simulink model "FOC_FZ"  (R2023b)
settings: Solver=FixedStepDiscrete  StartTime=0.0  StopTime=5  FixedStep=0.000001  RelTol=1e-3
libraries: simulink x2, spsDCVoltageSourceLib x1, spsPermanentMagnetSynchronousMachineLib x1, spsTwoLevelConverterLib x1, sps_lib x1
settings Model: Creator=LQY  LastModifiedBy=LQY

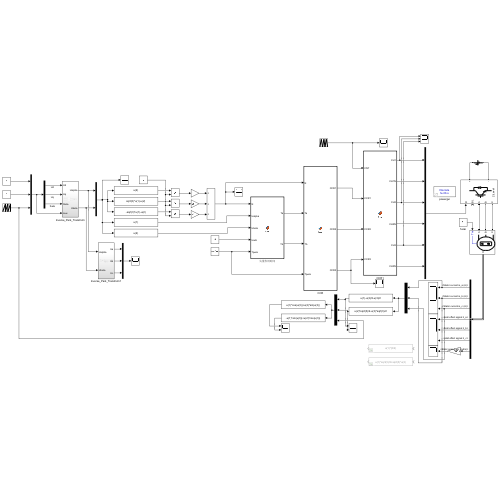
[thumbnail: Simulink's stored preview of the top-level diagram]
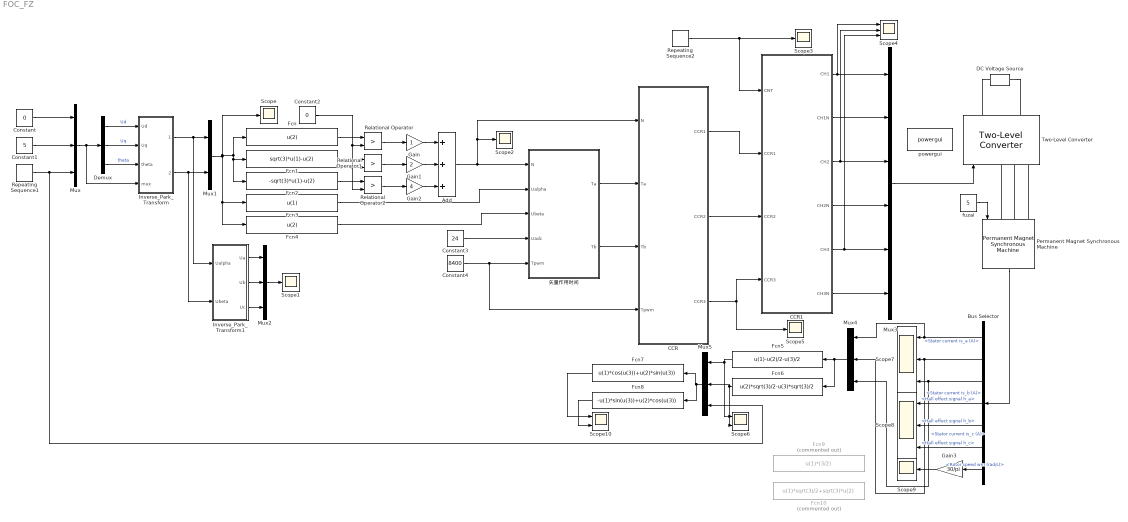
== system FOC_FZ ==
  Add : Sum  Inputs=+++
  Bus Selector : BusSelector  OutputSignals=Stator current is_a (A),Stator current is_b (A),Stator current is_c (A),Hall effect signal h_a,Hall effect signal h_b,Hall effect signal h_c,Rotor speed wm (rad/s)
  CCR : MATLAB Function  TreatAsAtomicUnit=on
  CCR1 : MATLAB Function  TreatAsAtomicUnit=on
  Constant : Constant  Value=0
  Constant1 : Constant  Value=5
  Constant2 : Constant  Value=0
  Constant3 : Constant  Value=24
  Constant4 : Constant  Value=8400
  DC Voltage Source : spsDCVoltageSourceLib/DC Voltage Source  Amplitude=24  Measurements=None
  Demux : Demux  Outputs=3
  Fcn : Fcn  Expr=u(2)
  Fcn1 : Fcn  Expr=sqrt(3)*u(1)-u(2)
  Fcn10 : Fcn  Commented=on  Expr=u(1)*sqrt(3)/2+sqrt(3)*u(2)
  Fcn2 : Fcn  Expr=-sqrt(3)*u(1)-u(2)
  Fcn3 : Fcn  Expr=u(1)
  Fcn4 : Fcn  Expr=u(2)
  Fcn5 : Fcn  Expr=u(1)-u(2)/2-u(3)/2
  Fcn6 : Fcn  Expr=u(2)*sqrt(3)/2-u(3)*sqrt(3)/2
  Fcn7 : Fcn  Expr=u(1)*cos(u(3))+u(2)*sin(u(3))
  Fcn8 : Fcn  Expr=-u(1)*sin(u(3))+u(2)*cos(u(3))
  Fcn9 : Fcn  Commented=on  Expr=u(1)*(3/2)
  Gain : Gain
  Gain1 : Gain  Gain=2
  Gain2 : Gain  Gain=4
  Gain3 : Gain  Gain=30/pi
  Inverse_Park_Transform : Subsystem
  Inverse_Park_Transform1 : Subsystem
  Mux{,2,4..5} (4 alike) : Mux  Inputs=3
  Mux1 : Mux  Inputs=2
  Mux3 : Mux  Inputs=6
  Permanent Magnet Synchronous Machine : spsPermanentMagnetSynchronousMachineLib/Permanent Magnet Synchronous Machine  NbPhases=3  FluxDistribution=Sinusoidal  RotorType=Round  MechanicalLoad=Torque Tm  PresetModel=No  ShowDetailedParameters=on  MeasurementBus=off  Resistance=0.0485  Inductance=8.5e-3  dqInductances=[8.5e-3,8.5e-3]  La=0.000395  MachineConstant=Flux linkage established by magnets (V.s)  Flux=0.1194  VoltageCst=43.3135  TorqueCst=0.3582  Flat=120  Mechanical=[0.0027 0.0004924 2 0]  PolePairs=4  InitialConditions=[0,0, 0,0]  InitialConditions5ph=[0 0 0 0 0 0]  RefAngle=Aligned with phase A axis (original Park)  IterativeDiscreteModel=Trapezoidal non iterative  TsBlock=-1  TsPowergui=0
  Relational Operator : RelationalOperator  Operator=>  OutDataTypeStr=boolean  RndMeth=Simplest  InputSameDT=off
  Relational Operator1 : RelationalOperator  Operator=>  OutDataTypeStr=boolean  RndMeth=Simplest  InputSameDT=off
  Relational Operator2 : RelationalOperator  Operator=>  OutDataTypeStr=boolean  RndMeth=Simplest  InputSameDT=off
  Repeating Sequence1 : simulink/Sources/Repeating Sequence  rep_seq_t=[0 0.5]  rep_seq_y=[0 2*pi]
  Repeating Sequence2 : simulink/Sources/Repeating Sequence  rep_seq_t=[0 0.00005 0.0001]  rep_seq_y=[0 4200 0]
  Scope{,1..3,5,9} (6 alike) : Scope
  Scope10 : Scope  NumInputPorts=2
  Scope4 : Scope  NumInputPorts=3
  Scope6 : Scope  NumInputPorts=2
  Scope7 : Scope  NumInputPorts=3
  Scope8 : Scope  NumInputPorts=3
  Two-Level Converter : spsTwoLevelConverterLib/Two-Level Converter  ModelType=Switching devices  Ron=1e-3  Rs=1e6  Cs=inf  Vforward=[0,0]  Ron_Diode=1e-3  Rs_Diode=1e6  Cs_Diode=inf  Vf_Diode=1e-3  Rs_CurrentSource=inf  Ron_ACsource=1e-3
      settings: LibrarySourceBlock=sps_lib/Power Electronics/Two-Level Converter
  fuzai : Constant  Value=5
  powergui : sps_lib/powergui  Priority=1  SimulationMode=Discrete  SampleTime=0.000001  frequency=60  Iterations=50  frequencyindice=0  Pbase=100e6  ErrMax=1e-4  UnitsV=kV  UnitsW=MW  buscounter=0  FunctionMessages=off  echomessages=off  EnableUseOfTLC=off  CurrentSourceSwitches=off  DisableSnubberDevices=off  DisableRonSwitches=off  DisableVfSwitches=off  DisplayEquations=off  AutomaticDiscreteSolvers=off  SolverType=Tustin/Backward Euler (TBE)  Interpol=off  ExternalGateDelay=off  methode=off  Ts=100  x0status=blocks  SPID=on  SwTol=0  HookPort=off  NonlinearTolerance=1e-4  nMaxIteration=100  ContinueOnMaxIteration=off  RestoreLinks=warning  ResistiveCurrentMeasurement=off  Frange=[0:2:500]  Ylog=off  Xlog=on  ShowGrid=off  save=off  variable=ZData  structure=0  ZoomFFT=off  StartTime=0.0  cycles=1  DisplayStyle=1  fundamental=60  FreqAxis=off  MaxFrequency=1000  frequencyindicesteady=1  RmsSteady=1  display=off
  矢量作用时间 : MATLAB Function  TreatAsAtomicUnit=on
  wires:
  Constant/1 -> Mux/1
  Constant1/1 -> Mux/2
  Repeating Sequence1/1 -> Mux5/3, Mux/3
  Mux/1 -> Inverse_Park_Transform/4(mux), Demux/1
  Mux1/1 -> Fcn2/1, Fcn1/1, Fcn/1, Scope/1, Fcn4/1, Fcn3/1
  Demux/1 -> Inverse_Park_Transform/1(Ud)  "Ud"
  Demux/2 -> Inverse_Park_Transform/2(Uq)  "Uq"
  Demux/3 -> Inverse_Park_Transform/3(theta)  "theta"
  Inverse_Park_Transform/1(Ualpha) -> Inverse_Park_Transform1/1(Ualpha), Mux1/1
  Inverse_Park_Transform/2(Ubeta) -> Mux1/2, Inverse_Park_Transform1/2(Ubeta)
  Inverse_Park_Transform1/2(Ub) -> Mux2/2
  Inverse_Park_Transform1/1(Ua) -> Mux2/1
  Inverse_Park_Transform1/3(Uc) -> Mux2/3
  Mux2/1 -> Scope1/1
  Fcn/1 -> Relational Operator/1
  Constant2/1 -> Relational Operator/2, Relational Operator1/2, Relational Operator2/2
  Fcn1/1 -> Relational Operator1/1
  Fcn2/1 -> Relational Operator2/1
  Relational Operator/1 -> Gain/1
  Relational Operator1/1 -> Gain1/1
  Relational Operator2/1 -> Gain2/1
  Gain/1 -> Add/1
  Gain1/1 -> Add/2
  Gain2/1 -> Add/3
  Add/1 -> 矢量作用时间/1(N), CCR/1(N), Scope2/1
  Fcn3/1 -> 矢量作用时间/2(Ualpha)
  Fcn4/1 -> 矢量作用时间/3(Ubeta)
  Constant3/1 -> 矢量作用时间/4(Uadc)
  Constant4/1 -> CCR/4(Tpwm), 矢量作用时间/5(Tpwm)
  矢量作用时间/1(Ta) -> CCR/2(Ta)
  矢量作用时间/2(Tb) -> CCR/3(Tb)
  Repeating Sequence2/1 -> CCR1/1(CNT), Scope3/1
  CCR/1(CCR1) -> CCR1/2(CCR1)
  CCR/2(CCR2) -> CCR1/3(CCR2)
  CCR/3(CCR3) -> Scope5/1, CCR1/4(CCR3)
  CCR1/6(CH3N) -> Mux3/6
  CCR1/5(CH3) -> Scope4/3, Mux3/5
  CCR1/4(CH2N) -> Mux3/4
  CCR1/3(CH2) -> Scope4/2, Mux3/3
  CCR1/2(CH1N) -> Mux3/2
  CCR1/1(CH1) -> Scope4/1, Mux3/1
  Mux3/1 -> Two-Level Converter/1
  fuzai/1 -> Permanent Magnet Synchronous Machine/1
  Permanent Magnet Synchronous Machine/1 -> Bus Selector/1
  Bus Selector/1 -> Mux4/1, Scope7/1  "<Stator current is_a (A)>"
  Bus Selector/2 -> Mux4/2, Scope7/2  "<Stator current is_b (A)>"
  Bus Selector/3 -> Mux4/3, Scope7/3  "<Stator current is_c (A)>"
  Bus Selector/4 -> Scope8/1  "<Hall effect signal h_a>"
  Bus Selector/5 -> Scope8/2  "<Hall effect signal h_b>"
  Bus Selector/6 -> Scope8/3  "<Hall effect signal h_c>"
  Bus Selector/7 -> Gain3/1  "<Rotor speed wm (rad/s)>"
  Gain3/1 -> Scope9/1
  Mux4/1 -> Fcn6/1, Fcn5/1
  Fcn5/1 -> Scope6/1, Mux5/1
  Fcn6/1 -> Scope6/2, Mux5/2
  Mux5/1 -> Fcn8/1, Fcn7/1
  Fcn7/1 -> Scope10/1
  Fcn8/1 -> Scope10/2
  connections:
  DC Voltage Source/RConn1 -- Two-Level Converter/RConn1
  DC Voltage Source/LConn1 -- Two-Level Converter/RConn2
  Permanent Magnet Synchronous Machine/LConn1 -- Two-Level Converter/LConn1
  Permanent Magnet Synchronous Machine/LConn2 -- Two-Level Converter/LConn2
  Permanent Magnet Synchronous Machine/LConn3 -- Two-Level Converter/LConn3

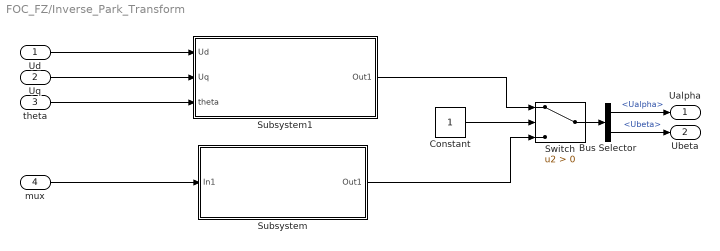
== system FOC_FZ/Inverse_Park_Transform ==
  Ud : Inport
  Uq : Inport  Port=2
  theta : Inport  Port=3
  mux : Inport  Port=4
  Bus Selector : BusSelector  OutputSignals=Ualpha,Ubeta
  Constant : Constant
  Subsystem : Subsystem
  Subsystem1 : Subsystem
  Switch : Switch  Criteria=u2 > Threshold  SaturateOnIntegerOverflow=off  InputSameDT=off
  Ualpha : Outport
  Ubeta : Outport  Port=2
  wires:
  Switch/1 -> Bus Selector/1
  Constant/1 -> Switch/2
  mux/1 -> Subsystem/1(In1)
  Subsystem/1(Out1) -> Switch/3
  Ud/1 -> Subsystem1/1(Ud)
  Uq/1 -> Subsystem1/2(Uq)
  theta/1 -> Subsystem1/3(theta)
  Subsystem1/1(Out1) -> Switch/1
  Bus Selector/2 -> Ubeta/1  "<Ubeta>"
  Bus Selector/1 -> Ualpha/1  "<Ualpha>"

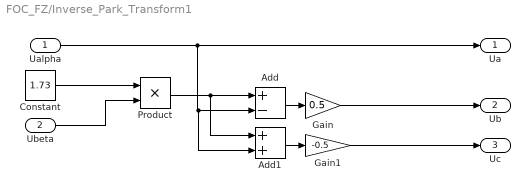
== system FOC_FZ/Inverse_Park_Transform1 ==
  Ualpha : Inport
  Ubeta : Inport  Port=2
  Add : Sum  Inputs=+-
  Add1 : Sum
  Constant : Constant  Value=1.73
  Gain : Gain  Gain=0.5
  Gain1 : Gain  Gain=-0.5
  Product : Product
  Ua : Outport
  Ub : Outport  Port=2
  Uc : Outport  Port=3
  wires:
  Ualpha/1 -> Add1/2, Add/2, Ua/1
  Constant/1 -> Product/1
  Ubeta/1 -> Product/2
  Product/1 -> Add1/1, Add/1
  Add/1 -> Gain/1
  Gain/1 -> Ub/1
  Add1/1 -> Gain1/1
  Gain1/1 -> Uc/1

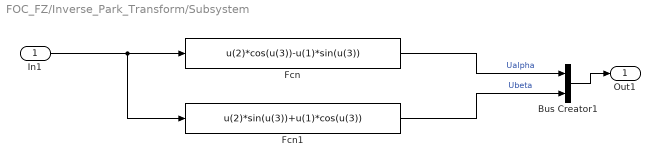
== system FOC_FZ/Inverse_Park_Transform/Subsystem ==
  In1 : Inport
  Bus Creator1 : BusCreator  Inputs=2
  Fcn : Fcn  Expr=u(2)*cos(u(3))-u(1)*sin(u(3))
  Fcn1 : Fcn  Expr=u(2)*sin(u(3))+u(1)*cos(u(3))
  Out1 : Outport
  wires:
  Fcn/1 -> Bus Creator1/1  "Ualpha"
  In1/1 -> Fcn1/1, Fcn/1
  Fcn1/1 -> Bus Creator1/2  "Ubeta"
  Bus Creator1/1 -> Out1/1

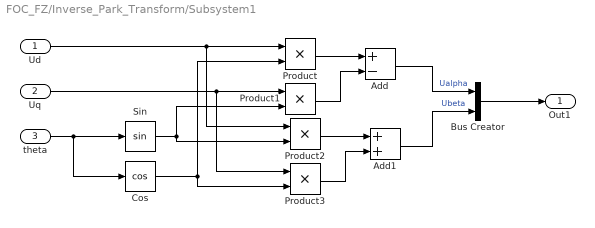
== system FOC_FZ/Inverse_Park_Transform/Subsystem1 ==
  Ud : Inport
  Uq : Inport  Port=2
  theta : Inport  Port=3
  Add : Sum  Inputs=+-
  Add1 : Sum
  Bus Creator : BusCreator  Inputs=2
  Cos : Trigonometry  Operator=cos
  Product{,1..3} (4 alike) : Product
  Sin : Trigonometry
  Out1 : Outport
  wires:
  Cos/1 -> Product3/2, Product/2
  Product3/1 -> Add1/2
  Sin/1 -> Product1/2, Product2/2
  theta/1 -> Sin/1, Cos/1
  Uq/1 -> Product3/1, Product1/1
  Ud/1 -> Product2/1, Product/1
  Product1/1 -> Add/2
  Product/1 -> Add/1
  Product2/1 -> Add1/1
  Add1/1 -> Bus Creator/2  "Ubeta"
  Add/1 -> Bus Creator/1  "Ualpha"
  Bus Creator/1 -> Out1/1

== matlab function FOC_FZ/CCR ==
  data: N input; CCR1 output; Ta input; Tb input; Tpwm input; CCR2 output; CCR3 output
function [CCR1,CCR2,CCR3] = fcn(N,Ta,Tb,Tpwm)

CCR1=double(0);
CCR2=double(0);
CCR3=double(0);

Temp=Ta+Tb;
if(Temp>Tpwm)
    Ta=Ta/Temp*Tpwm;
    Tb=Tb/Temp*Tpwm;
end

value1=(Tpwm-Ta-Tb)/4.0;
value2=value1+Ta/2.0;
value3=value2+Tb/2.0;

switch(N)
    case 3
        CCR1=value1;
        CCR2=value2;
        CCR3=value3;
    case 1
        CCR1=value2;
        CCR2=value1;
        CCR3=value3;
    case 5
        CCR1=value3;
        CCR2=value1;
        CCR3=value2;
    case 4
        CCR1=value3;
        CCR2=value2;
        CCR3=value1;
    case 6
        CCR1=value2;
        CCR2=value3;
        CCR3=value1;
    case 2
        CCR1=value1;
        CCR2=value3;
        CCR3=value2;
end

== matlab function FOC_FZ/矢量作用时间 ==
  data: N input; Ta output; Ualpha input; Ubeta input; Uadc input; Tpwm input; Tb output
function [Ta,Tb] = fcn(N,Ualpha,Ubeta,Uadc,Tpwm)

Ta=double(0);
Tb=double(0);
X=(sqrt(3)*Tpwm)/Uadc*Ubeta;            %系数1 
Y=(sqrt(3)*Tpwm)/Uadc*((sqrt(3)/2)*Ualpha-(1/2)*Ubeta);  %系数2
Z=(sqrt(3)*Tpwm)/Uadc*(-(sqrt(3)/2)*Ualpha-(1/2)*Ubeta);   %系数3
    
if(N==3)   %第一扇区
   Ta=Y;
   Tb=X;
end
if(N==1)   %第二扇区
   Ta=-Y;
   Tb=-Z;
end
if(N==5)   %第三扇区
   Ta=X;
   Tb=Z;
end
if(N==4)   %第四扇区
   Ta=-X;
   Tb=-Y;
end
if(N==6)   %第五扇区
   Ta=Z;
   Tb=Y;
end
if(N==2)   %第六扇区
   Ta=-Z;
   Tb=-X;
end

== matlab function FOC_FZ/CCR1 ==
  data: CNT input; CH1 output; CCR1 input; CCR2 input; CCR3 input; CH1N output; CH2 output; CH2N output; CH3 output; CH3N output
function [CH1,CH1N,CH2,CH2N,CH3,CH3N] = fcn(CNT,CCR1,CCR2,CCR3)

if(CNT<CCR1)
  CH1=0;
  CH1N=1;
else
  CH1=1;
  CH1N=0;   
end
if(CNT<CCR2)
  CH2=0;
  CH2N=1;
 else
  CH2=1;
  CH2N=0;  
end
if(CNT<CCR3)
  CH3=0;
  CH3N=1;
else
  CH3=1;
  CH3N=0;  
end
